simulink model "Pacemaker_images"  (R2022a)
settings: Solver=FixedStepAuto  StartTime=0.0  StopTime=40  FixedStep=1e-3  RelTol=1e-3  EnableMultiTasking=on
undefined symbols (not defined in the file or in its folder): ARP, ATR_Amplitude, ATR_CMP_DETECT, ATR_Pulse_Width, ATR_Sensitivity, D10, D11, D12, D13, D2, D3, D4, D5, D6, D7, D8, D9, Flag, Hecate_delayEnd, Hecate_delayOff, Hecate_delayOn, LRL, Mode, PTA0, PTA1, PTA2, PTB23, PTB9, PTC2, PTC3, PTC4, PTD0, PTD1, PTD2, PTD3, VENT_Amplitude, VENT_CMP_DETECT, VENT_PACE_CTRL, VENT_Pulse_Width, VENT_Sensitivity, VRP
libraries: frdmk64flib x15
settings Model: ExtModeTrigDuration=5  Creator=akshayjacob  LastModifiedBy=fedformi_new
settings DataIOCC: SaveFormat=Array  ReturnWorkspaceOutputs=off
settings OptimizationCC: DefaultParameterBehavior=Inlined  EnhancedBackFolding=on  PassReuseOutputArgsAs=Individual arguments  ZeroExternalMemoryAtStartup=off  ZeroInternalMemoryAtStartup=off  MaxStackSize=64  OptimizeBlockOrder=speed  DifferentSizesBufferReuse=on  OptimizationCustomize=off  EfficientTunableParamExpr=on
settings DebuggingCC: ParameterTunabilityLossMsg=error  UnconnectedInputMsg=warning  UnconnectedOutputMsg=warning  UnconnectedLineMsg=warning
settings HardwareCC: ProdBitPerPointer=32  ProdBitPerSizeT=32  ProdBitPerPtrDiffT=32  ProdLargestAtomicInteger=Long  ProdLargestAtomicFloat=Double  ProdWordSize=32  ProdHWDeviceType=ARM Compatible->ARM Cortex
settings SFSimCC: MATLABDynamicMemAlloc=off
settings RTWCC: SystemTargetFile=ert.tlc  TemplateMakefile=ert_default_tmf  Toolchain=GNU Tools for ARM Embedded Processors  DLArmComputeVersion=19.05
settings CodeAppCC: ForceParamTrailComments=on  IgnoreCustomStorageClasses=off  OperatorAnnotations=on  SimulinkDataObjDesc=on  SFDataObjDesc=on  InsertBlockDesc=on
settings ERTTargetCC: ERTCustomFileTemplate=example_file_process.tlc

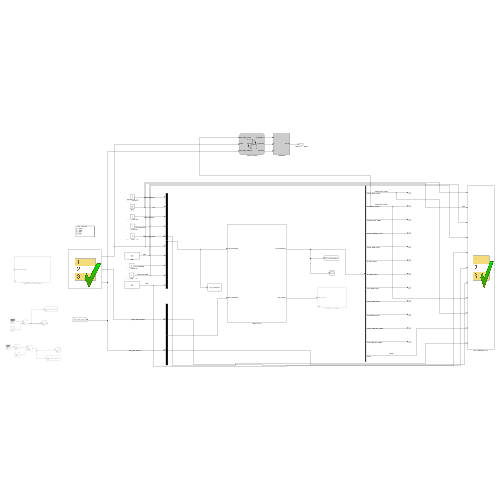
[thumbnail: Simulink's stored preview of the top-level diagram]
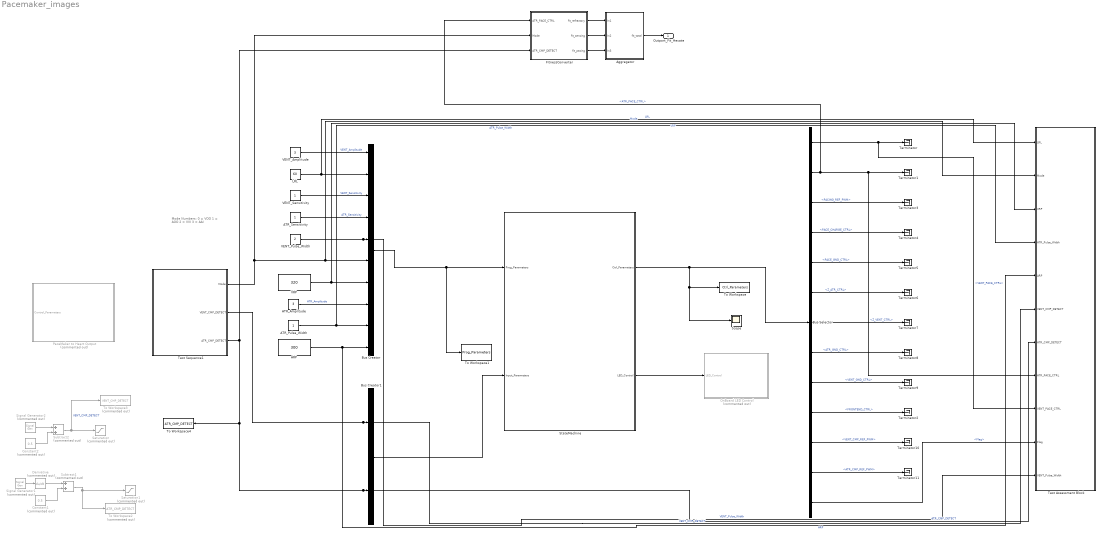
== system Pacemaker_images ==
  note: Mode Numbers:
      |
      | 0 = VOO
      | 1 = AOO
      | 2 = VVI
      | 3 = AAI
  ARP : Constant  Value=300
  ATR_Amplitude : Constant  Value=3
  ATR_Pulse_Width : Constant
  ATR_Sensitivity : Constant
  Aggregator : Subsystem
  Bus Creator : BusCreator  Inputs=VENT_Amplitude,LRL,VENT_Sensitivity,ATR_Sensitivity,VENT_Pulse_Width,Mode,VRP,ATR_Amplitude,ATR_Pulse_Width,ARP
  Bus Creator1 : BusCreator  Inputs=VENT_CMP_DETECT,ATR_CMP_DETECT
  Bus Selector : BusSelector  OutputSignals=VENT_PACE_CTRL,ATR_PACE_CTRL,PACING_REF_PWM,PACE_CHARGE_CTRL,PACE_GND_CTRL,Z_ATR_CTRL,Z_VENT_CTRL,ATR_GND_CTRL,VENT_GND_CTRL,FRONTEND_CTRL,VENT_CMP_REF_PWM,ATR_CMP_REF_PWM,Flag
  Constant1 : Constant  Commented=on  Value=0.5
  Constant2 : Constant  Commented=on  Value=0.5
  Derivative : Derivative  Commented=on
  FitnessConverter : Stateflow chart  TreatAsAtomicUnit=on
  LRL : Constant  Value=60
  OnBoard LED Control : Subsystem  Commented=on
  PaceMaker to Heart Output : Subsystem  Commented=on
  Saturation : Saturate  Commented=on  UpperLimit=1  LowerLimit=0
  Saturation1 : Saturate  Commented=on  UpperLimit=1  LowerLimit=0
  Scope : Scope
  Signal Generator1 : SignalGenerator  Commented=on  Amplitude=1.5  Frequency=1/5
  Signal Generator2 : SignalGenerator  Commented=on  Amplitude=1.5  Frequency=1/5
  StateMachine : Subsystem
  Subtract1 : Sum  Commented=on
  Subtract2 : Sum  Commented=on
  Terminator{,1..11} (12 alike) : Terminator
  Test Assessment Block : Test Sequence  Tag=__SLT_ASMT__  TreatAsAtomicUnit=on
  Test Sequence1 : Test Sequence  TreatAsAtomicUnit=on
  To Workspace : ToWorkspace  VariableName=Ctrl_Parameters  SaveFormat=Timeseries  SampleTime=-1
  To Workspace1 : ToWorkspace  VariableName=Prog_Parameters  SaveFormat=Timeseries  SampleTime=-1
  To Workspace2 : ToWorkspace  Commented=on  VariableName=ATR_CMP_DETECT  SaveFormat=Timeseries  SampleTime=-1
  To Workspace3 : ToWorkspace  Commented=on  VariableName=VENT_CMP_DETECT  SaveFormat=Timeseries  SampleTime=-1
  To Workspace4 : ToWorkspace  VariableName=ATR_CMP_DETECT  SaveFormat=Timeseries  SampleTime=-1
  VENT_Amplitude : Constant  Value=3
  VENT_Pulse_Width : Constant  Value=2
  VENT_Sensitivity : Constant
  VRP : Constant  Value=320
  Outport_Fit_Hecate : Outport
  wires:
  Bus Creator/1 -> To Workspace1/1, StateMachine/1(Prog_Parameters)
  StateMachine/2(LED_Control) -> OnBoard LED Control/1(LED_Control)
  Bus Creator1/1 -> StateMachine/2(Input_Parameters)
  VRP/1 -> Bus Creator/7, Test Assessment Block/3(VRP)  "VRP"
  ATR_Sensitivity/1 -> Bus Creator/4  "ATR_Sensitivity"
  ATR_Pulse_Width/1 -> Bus Creator/9, Test Assessment Block/4(ATR_Pulse_Width)  "ATR_Pulse_Width"
  LRL/1 -> Bus Creator/2, Test Assessment Block/1(LRL)  "LRL"
  ATR_Amplitude/1 -> Bus Creator/8  "ATR_Amplitude"
  ARP/1 -> Bus Creator/10, Test Assessment Block/5(ARP)  "ARP"
  VENT_Sensitivity/1 -> Bus Creator/3  "VENT_Sensitivity"
  VENT_Amplitude/1 -> Bus Creator/1  "VENT_Amplitude"
  VENT_Pulse_Width/1 -> Test Assessment Block/11(VENT_Pulse_Width), Bus Creator/5  "VENT_Pulse_Width"
  Test Sequence1/1(Mode) -> Test Assessment Block/2(Mode), Bus Creator/6, FitnessConverter/2(Mode)  "Mode"
  Subtract1/1 -> Saturation1/1, To Workspace2/1
  Signal Generator2/1 -> Subtract2/1
  Test Sequence1/2(VENT_CMP_DETECT) -> Test Assessment Block/6(VENT_CMP_DETECT), Bus Creator1/1  "VENT_CMP_DETECT"
  Constant1/1 -> Subtract1/2
  Constant2/1 -> Subtract2/2
  Test Sequence1/3(ATR_CMP_DETECT) -> FitnessConverter/3(ATR_CMP_DETECT), To Workspace4/1, Test Assessment Block/7(ATR_CMP_DETECT), Bus Creator1/2  "ATR_CMP_DETECT"
  Subtract2/1 -> Saturation/1, To Workspace3/1  "VENT_CMP_DETECT"
  Derivative/1 -> Subtract1/1
  Signal Generator1/1 -> Derivative/1
  Bus Selector/12 -> Terminator11/1  "<ATR_CMP_REF_PWM>"
  Bus Selector/3 -> Terminator3/1  "<PACING_REF_PWM>"
  Bus Selector/7 -> Terminator7/1  "<Z_VENT_CTRL>"
  Bus Selector/10 -> Terminator2/1  "<FRONTEND_CTRL>"
  Bus Selector/8 -> Terminator8/1  "<ATR_GND_CTRL>"
  StateMachine/1(Ctrl_Parameters) -> Bus Selector/1, Scope/1, To Workspace/1
  Bus Selector/1 -> Test Assessment Block/9(VENT_PACE_CTRL), Terminator/1  "<VENT_PACE_CTRL>"
  Bus Selector/5 -> Terminator5/1  "<PACE_GND_CTRL>"
  Bus Selector/9 -> Terminator9/1  "<VENT_GND_CTRL>"
  Bus Selector/2 -> Test Assessment Block/8(ATR_PACE_CTRL), Terminator1/1, FitnessConverter/1(ATR_PACE_CTRL)  "<ATR_PACE_CTRL>"
  Bus Selector/11 -> Terminator10/1  "<VENT_CMP_REF_PWM>"
  Bus Selector/6 -> Terminator6/1  "<Z_ATR_CTRL>"
  Bus Selector/4 -> Terminator4/1  "<PACE_CHARGE_CTRL>"
  Bus Selector/13 -> Test Assessment Block/10(Flag)  "<Flag>"
  FitnessConverter/1(fit_refractory) -> Aggregator/1(In1)
  FitnessConverter/2(fit_sensing) -> Aggregator/2(In2)
  FitnessConverter/3(fit_pacing) -> Aggregator/3(In3)
  Aggregator/1(fit_total) -> Outport_Fit_Hecate/1

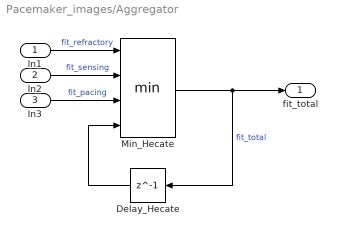
== system Pacemaker_images/Aggregator ==
  In1 : Inport
  In2 : Inport  Port=2
  In3 : Inport  Port=3
  Delay_Hecate : Delay  DelayLength=1  InitialCondition=Inf
  Min_Hecate : MinMax  Inputs=4
  fit_total : Outport
  wires:
  In2/1 -> Min_Hecate/2  "fit_sensing"
  In3/1 -> Min_Hecate/3  "fit_pacing"
  Delay_Hecate/1 -> Min_Hecate/4
  In1/1 -> Min_Hecate/1  "fit_refractory"
  Min_Hecate/1 -> fit_total/1, Delay_Hecate/1  "fit_total"

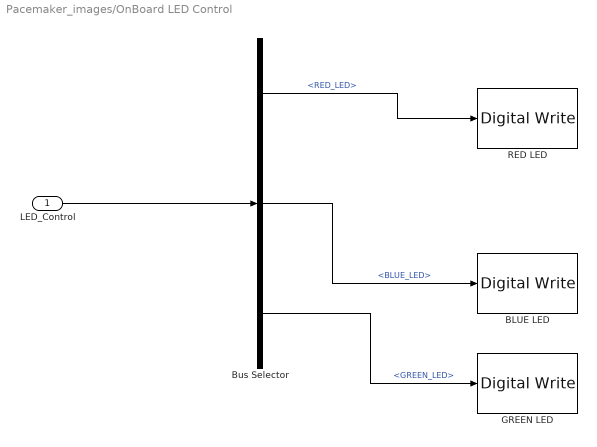
== system Pacemaker_images/OnBoard LED Control ==
  LED_Control : Inport
  BLUE LED : frdmk64flib/Digital Write  Whichpin=BLUE_LED
  Bus Selector : BusSelector  OutputSignals=RED_LED,BLUE_LED,GREEN_LED
  GREEN LED : frdmk64flib/Digital Write  Whichpin=GREEN_LED
  RED LED : frdmk64flib/Digital Write  Whichpin=RED_LED
  wires:
  LED_Control/1 -> Bus Selector/1
  Bus Selector/1 -> RED LED/1  "<RED_LED>"
  Bus Selector/2 -> BLUE LED/1  "<BLUE_LED>"
  Bus Selector/3 -> GREEN LED/1  "<GREEN_LED>"

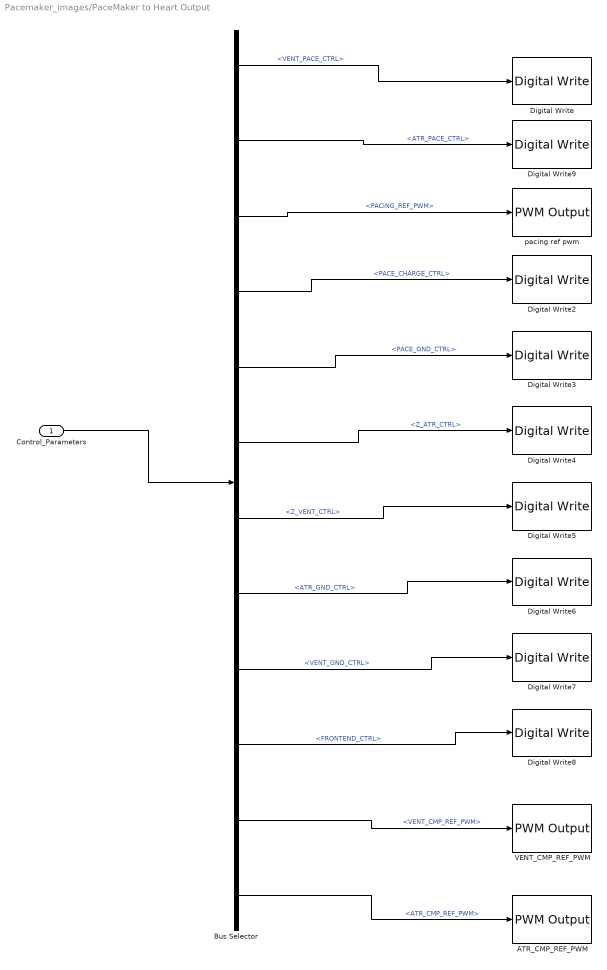
== system Pacemaker_images/PaceMaker to Heart Output ==
  Control_Parameters : Inport
  ATR_CMP_REF_PWM : frdmk64flib/PWM Output  Whichpin=PTC2 (D6)  InitialFrequency=2000  InitialDutyCycle=0
  Bus Selector : BusSelector  OutputSignals=VENT_PACE_CTRL,ATR_PACE_CTRL,PACING_REF_PWM,PACE_CHARGE_CTRL,PACE_GND_CTRL,Z_ATR_CTRL,Z_VENT_CTRL,ATR_GND_CTRL,VENT_GND_CTRL,FRONTEND_CTRL,VENT_CMP_REF_PWM,ATR_CMP_REF_PWM
  Digital Write : frdmk64flib/Digital Write  Whichpin=PTC4 (D9)
  Digital Write2 : frdmk64flib/Digital Write  Whichpin=PTB9 (D2)
  Digital Write3 : frdmk64flib/Digital Write  Whichpin=PTD0 (D10)
  Digital Write4 : frdmk64flib/Digital Write  Whichpin=PTB23 (D4)
  Digital Write5 : frdmk64flib/Digital Write  Whichpin=PTC3 (D7)
  Digital Write6 : frdmk64flib/Digital Write  Whichpin=PTD2 (D11)
  Digital Write7 : frdmk64flib/Digital Write  Whichpin=PTD3 (D12)
  Digital Write8 : frdmk64flib/Digital Write  Whichpin=PTD1 (D13)
  Digital Write9 : frdmk64flib/Digital Write  Whichpin=PTA0 (D8)
  VENT_CMP_REF_PWM : frdmk64flib/PWM Output  Whichpin=PTA1 (D3)  InitialFrequency=2000  InitialDutyCycle=0
  pacing ref pwm : frdmk64flib/PWM Output  Whichpin=PTA2 (D5)  InitialFrequency=2000  InitialDutyCycle=0
  wires:
  Control_Parameters/1 -> Bus Selector/1
  Bus Selector/1 -> Digital Write/1  "<VENT_PACE_CTRL>"
  Bus Selector/3 -> pacing ref pwm/1  "<PACING_REF_PWM>"
  Bus Selector/4 -> Digital Write2/1  "<PACE_CHARGE_CTRL>"
  Bus Selector/5 -> Digital Write3/1  "<PACE_GND_CTRL>"
  Bus Selector/6 -> Digital Write4/1  "<Z_ATR_CTRL>"
  Bus Selector/7 -> Digital Write5/1  "<Z_VENT_CTRL>"
  Bus Selector/8 -> Digital Write6/1  "<ATR_GND_CTRL>"
  Bus Selector/9 -> Digital Write7/1  "<VENT_GND_CTRL>"
  Bus Selector/10 -> Digital Write8/1  "<FRONTEND_CTRL>"
  Bus Selector/2 -> Digital Write9/1  "<ATR_PACE_CTRL>"
  Bus Selector/11 -> VENT_CMP_REF_PWM/1  "<VENT_CMP_REF_PWM>"
  Bus Selector/12 -> ATR_CMP_REF_PWM/1  "<ATR_CMP_REF_PWM>"

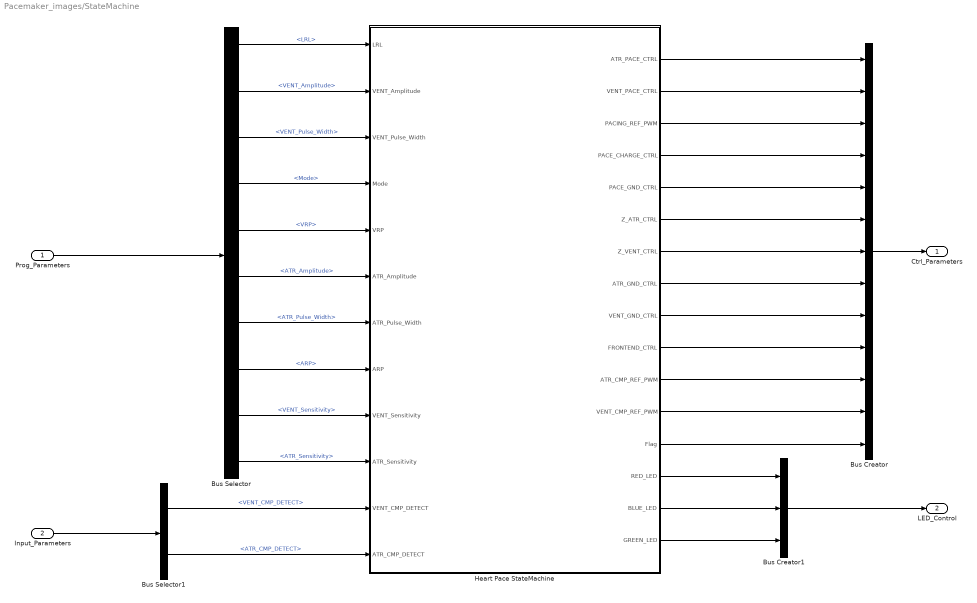
== system Pacemaker_images/StateMachine ==
  Prog_Parameters : Inport
  Input_Parameters : Inport  Port=2
  Bus Creator : BusCreator  Inputs=13
  Bus Creator1 : BusCreator  Inputs=3
  Bus Selector : BusSelector  OutputSignals=LRL,VENT_Amplitude,VENT_Pulse_Width,Mode,VRP,ATR_Amplitude,ATR_Pulse_Width,ARP,VENT_Sensitivity,ATR_Sensitivity
  Bus Selector1 : BusSelector  OutputSignals=VENT_CMP_DETECT,ATR_CMP_DETECT
  Heart Pace StateMachine : Stateflow chart  TreatAsAtomicUnit=on
      settings: PortSchema="{\"entries\":[{\"content\":{\"sides\":[{\"content\":{\"connectorIds\":[\"In1\",\"In2\",\"In3\",\"In4\",\"In5\",\"In6\",\"In7\",\"In8\",\"In9\",\"In10\",\"In11\",\"In12\"]},\"type\":\"ConnectorPlacement.EquallySpacedRectSide\",\"uuid\":\"078f44e2-9792-46c6-9fab-c05fe0916fc5\"},{\"content\":{\"connectorIds\":[\"Out1\",\"Out2\",\"Out3\",\"Out4\",\"Out5\",\"Out6\",\"Out7\",\"Out8\",\"Out9\",\"Out10\",\"Out14\",\"Out15\",\"Out16\",\"Out11\",\"Out12\",\"Out13\"],\"side\":\"RIGHT\"},\"type\":\"ConnectorPlacement.EquallySpacedRectSide\",\"uuid\":\"2df68980-2ea6-42d1-b726-b24978220bfa\"},{\"content\":{\"connectorIds\":[],\"side\":\"TOP\"},\"type\":\"ConnectorPlacement.EquallySpacedRectSide\",\"uuid\":\"4f99418a-e276-4e4c-8fb0-96ffb017fecf\"}]},\"type\":\"ConnectorPlacement.EquallySpacedConnector\",\"uuid\":\"ac4267e7-732c-486f-b9a5-28cca0f40ec4\"}],\"packageUris\":[\"http://schema.mathworks.com/mf0/Connector/R2020b\"],\"version\":\"1.0\"}"
  Ctrl_Parameters : Outport
  LED_Control : Outport  Port=2
  wires:
  Prog_Parameters/1 -> Bus Selector/1
  Bus Selector/1 -> Heart Pace StateMachine/1(LRL)  "<LRL>"
  Bus Selector/2 -> Heart Pace StateMachine/2(VENT_Amplitude)  "<VENT_Amplitude>"
  Bus Selector/3 -> Heart Pace StateMachine/3(VENT_Pulse_Width)  "<VENT_Pulse_Width>"
  Bus Selector/4 -> Heart Pace StateMachine/4(Mode)  "<Mode>"
  Heart Pace StateMachine/1(ATR_PACE_CTRL) -> Bus Creator/1
  Heart Pace StateMachine/2(VENT_PACE_CTRL) -> Bus Creator/2
  Bus Creator/1 -> Ctrl_Parameters/1
  Heart Pace StateMachine/3(PACING_REF_PWM) -> Bus Creator/3
  Heart Pace StateMachine/4(PACE_CHARGE_CTRL) -> Bus Creator/4
  Heart Pace StateMachine/5(PACE_GND_CTRL) -> Bus Creator/5
  Heart Pace StateMachine/6(Z_ATR_CTRL) -> Bus Creator/6
  Heart Pace StateMachine/7(Z_VENT_CTRL) -> Bus Creator/7
  Heart Pace StateMachine/8(ATR_GND_CTRL) -> Bus Creator/8
  Heart Pace StateMachine/9(VENT_GND_CTRL) -> Bus Creator/9
  Heart Pace StateMachine/10(FRONTEND_CTRL) -> Bus Creator/10
  Heart Pace StateMachine/11(RED_LED) -> Bus Creator1/1
  Heart Pace StateMachine/12(BLUE_LED) -> Bus Creator1/2
  Bus Creator1/1 -> LED_Control/1
  Heart Pace StateMachine/13(GREEN_LED) -> Bus Creator1/3
  Input_Parameters/1 -> Bus Selector1/1
  Bus Selector1/1 -> Heart Pace StateMachine/11(VENT_CMP_DETECT)  "<VENT_CMP_DETECT>"
  Bus Selector1/2 -> Heart Pace StateMachine/12(ATR_CMP_DETECT)  "<ATR_CMP_DETECT>"
  Bus Selector/6 -> Heart Pace StateMachine/6(ATR_Amplitude)  "<ATR_Amplitude>"
  Bus Selector/7 -> Heart Pace StateMachine/7(ATR_Pulse_Width)  "<ATR_Pulse_Width>"
  Bus Selector/8 -> Heart Pace StateMachine/8(ARP)  "<ARP>"
  Bus Selector/9 -> Heart Pace StateMachine/9(VENT_Sensitivity)  "<VENT_Sensitivity>"
  Bus Selector/10 -> Heart Pace StateMachine/10(ATR_Sensitivity)  "<ATR_Sensitivity>"
  Heart Pace StateMachine/14(ATR_CMP_REF_PWM) -> Bus Creator/11
  Heart Pace StateMachine/15(VENT_CMP_REF_PWM) -> Bus Creator/12
  Bus Selector/5 -> Heart Pace StateMachine/5(VRP)  "<VRP>"
  Heart Pace StateMachine/16(Flag) -> Bus Creator/13

== stateflow chart Pacemaker_images/Test Assessment Block ==
  state Run
    state AAI
      state AAI_Refractory
        verify(ATR_PACE_CTRL==0)
      state AAI_Sensing
        verify(ATR_PACE_CTRL==0)
      state AAI_Pacing
        verify(ATR_PACE_CTRL==1);
      (default) -> AAI_Refractory
      (junction 475) -> AAI_Refractory
      (junction 494) -> (junction 475)
      AAI_Refractory -> AAI_Sensing : [
          | after(ARP-(ATR_Pulse_Width ...
          | *Flag),msec)
          | ]
      AAI_Sensing -> AAI_Refractory [order 1] : [
          | [(ATR_CMP_DETECT == 1)]
          | ]
      AAI_Sensing -> AAI_Pacing [order 2] : [
          | after(60000/LRL-ARP, msec)
          | ]
      AAI_Pacing -> (junction 494) : [
          | after(ATR_Pulse_Width,msec)
          | ]
    state VVI
      state VVI_REFRACTORY
        verify(VENT_PACE_CTRL==0);
      state VVI_SENSE
        verify(VENT_PACE_CTRL==0);
      state VVI_PACING
        verify(VENT_PACE_CTRL==1);
      (junction 541) -> (junction 535)
      (default) -> VVI_REFRACTORY
      (junction 535) -> VVI_REFRACTORY
      VVI_REFRACTORY -> VVI_SENSE : [
          | after(VRP - (VENT_Pulse_Width * Flag-1),msec)
          | ]
      VVI_SENSE -> VVI_REFRACTORY [order 2] : [
          | VENT_CMP_DETECT == 1
          | ]
      VVI_SENSE -> VVI_PACING [order 1] : [
          | after(60000/LRL - VRP, msec)
          | ]
      VVI_PACING -> (junction 541) : [
          | after(VENT_Pulse_Width,msec)
          | ]
    state default
    (junction 517) -> (junction 520) [order 2]
    (junction 407) -> (junction 516) [order 2]
    Run -> (junction 407)
    (junction 407) -> (junction 390) [order 1] : [Mode == 3
        | ]
    (junction 516) -> (junction 418) [order 2]
    (junction 390) -> AAI [order 1] : [~in(Run.AAI)]
    (junction 390) -> (junction 393) [order 2]
    (default) -> (junction 407)
    (junction 516) -> (junction 517) [order 1] : [Mode ==2
        | ]
    (junction 517) -> VVI [order 1] : [~in(Run.VVI)]
    (junction 418) -> (junction 419)
    (junction 419) -> default [order 1] : [~in(Run.default)]
    (junction 419) -> (junction 422) [order 2]
  (default) -> Run
  data: LRL input double size=[1]; Mode input double size=[1]; VRP input size=[1]; ATR_Pulse_Width input double size=[1]; ARP input size=[1]; VENT_CMP_DETECT input size=[1, 1]; ATR_CMP_DETECT input size=[1, 1]; ATR_PACE_CTRL input double size=[1]; VENT_PACE_CTRL input double size=[1]; Flag input; VENT_Pulse_Width input

== stateflow chart Pacemaker_images/Test Sequence1 ==
  settings: updateMethod=DISCRETE  sampleTime=0.001
  state Initialize
    %. . .
    ATR_CMP_DETECT=false;
  state AAI_Mode_3
    Mode=3;
    state AAI_Mode_3_OFF
      ATR_CMP_DETECT=false;
    state AAI_Mode_3_ON
      ATR_CMP_DETECT=true;
    (default) -> AAI_Mode_3_OFF
    AAI_Mode_3_OFF -> AAI_Mode_3_ON : [
        | after(3+...
        | Hecate_delayOn,sec)
        | ]
    AAI_Mode_3_ON -> AAI_Mode_3_OFF : [
        | after(1+...
        | Hecate_delayOff,sec)
        | ]
  state END
    ATR_CMP_DETECT=false;
  (default) -> Initialize
  Initialize -> AAI_Mode_3 : [
      | true
      | ]
  AAI_Mode_3 -> END : [
      | after(20+...
      | Hecate_delayEnd,sec)
      | ]
  data: Mode output double size=[1]; VENT_CMP_DETECT output boolean size=[1, 1]; ATR_CMP_DETECT output boolean size=[1, 1]; Hecate_delayEnd parameter; Hecate_delayOn parameter; Hecate_delayOff parameter

== stateflow chart Pacemaker_images/FitnessConverter ==
  state Run
    fit_refractory = Inf;
    fit_sensing = Inf;
    fit_pacing = Inf;
    state default
      fit_refractory = Inf;
      fit_sensing = Inf;
      fit_pacing = Inf;
    state AAI
      fit_refractory = Inf;
      fit_sensing = Inf;
      fit_pacing = Inf;
      state AAI_Refractory
        fit_refractory = ...
        abs(ATR_PACE_CTRL-(0));
        fit_sensing = Inf;
        fit_pacing = Inf;
      state AAI_Sensing
        fit_refractory = Inf;
        fit_sensing = ...
        abs(ATR_PACE_CTRL-(0));
        fit_pacing = Inf;
      state AAI_Pacing
        fit_refractory = Inf;
        fit_sensing = Inf;
        fit_pacing = ...
        abs(ATR_PACE_CTRL-(1));
      AAI_Sensing -> AAI_Refractory [order 1] : [[(ATR_CMP_DETECT == 1)]]
      (default) -> AAI_Refractory
      AAI_Refractory -> AAI_Sensing : [after(ARP-(ATR_Pulse_Width ...
          | *Flag),msec)]
      AAI_Sensing -> AAI_Pacing [order 2] : [after(60000/LRL-ARP, msec)]
      AAI_Pacing -> AAI_Refractory : [after(ATR_Pulse_Width,msec)]
    state VVI
      fit_refractory = Inf;
      fit_sensing = Inf;
      fit_pacing = Inf;
      state VVI_REFRACTORY
        fit_refractory = Inf;
        fit_sensing = Inf;
        fit_pacing = Inf;
      state VVI_SENSE
        fit_refractory = Inf;
        fit_sensing = Inf;
        fit_pacing = Inf;
      state VVI_PACING
        fit_refractory = Inf;
        fit_sensing = Inf;
        fit_pacing = Inf;
      (default) -> VVI_REFRACTORY
      VVI_SENSE -> VVI_REFRACTORY [order 2] : [VENT_CMP_DETECT == 1]
      VVI_PACING -> VVI_REFRACTORY : [after(VENT_Pulse_Width,msec)]
      VVI_SENSE -> VVI_PACING [order 1] : [after(60000/LRL - VRP, msec)]
      VVI_REFRACTORY -> VVI_SENSE : [after(VRP - (VENT_Pulse_Width * Flag-1),msec)]
    default -> (junction 48) : [(Mode==2)|(Mode==3)]
    (default) -> (junction 48)
    (junction 48) -> default [order 3]
    AAI -> (junction 48) : [~(Mode==2)]
    (junction 48) -> VVI [order 2] : [Mode==3]
    VVI -> (junction 48) : [(Mode==2)|~(Mode==3)]
    (junction 48) -> AAI [order 1] : [Mode==2]
  (default) -> Run
  data: fit_refractory output; ATR_PACE_CTRL input; Mode input; LRL parameter; VRP parameter; ATR_Pulse_Width parameter; ARP parameter; VENT_CMP_DETECT parameter; VENT_PACE_CTRL parameter; Flag parameter; VENT_Pulse_Width parameter; fit_sensing output; fit_pacing output; ATR_CMP_DETECT input

== stateflow chart Pacemaker_images/StateMachine/Heart Pace StateMachine ==
  state VOO_ChargingState
    entry:
    ATR_PACE_CTRL = 0;
    VENT_PACE_CTRL = 0;
    PACING_REF_PWM = VENT_Amplitude/5*100
    PACE_CHARGE_CTRL = 1;
    PACE_GND_CTRL = 1;
    Z_ATR_CTRL = 0;
    Z_VENT_CTRL = 0;
    ATR_GND_CTRL = 0;
    VENT_GND_CTRL = 1;
    BLUE_LED = 0;
    RED_LED = 1;
  state VOO_Pacing
    entry:
    PACE_CHARGE_CTRL = 0;
    PACE_GND_CTRL = 1;
    ATR_GND_CTRL = 0;
    ATR_PACE_CTRL = 0;
    Z_ATR_CTRL = 0;
    Z_VENT_CTRL =0;
    VENT_PACE_CTRL = 1;
    VENT_GND_CTRL = 0;
    PACING_REF_PWM = VENT_Amplitude/5*100;
    BLUE_LED=1;
    RED_LED=0;
  state AOO_ChargingState
    entry:
    ATR_PACE_CTRL = 0;
    VENT_PACE_CTRL = 0;
    PACING_REF_PWM = ATR_Amplitude/5*100
    PACE_CHARGE_CTRL = 1;
    PACE_GND_CTRL = 1;
    Z_ATR_CTRL = 0;
    Z_VENT_CTRL = 0;
    ATR_GND_CTRL = 1;
    VENT_GND_CTRL = 0;
    BLUE_LED = 0;
    RED_LED = 1;
  state AOO_Pacing
    entry:
    PACE_CHARGE_CTRL = 0;
    PACE_GND_CTRL = 1;
    ATR_GND_CTRL = 0;
    ATR_PACE_CTRL = 1;
    Z_ATR_CTRL = 0;
    Z_VENT_CTRL =0;
    VENT_PACE_CTRL = 0;
    VENT_GND_CTRL = 0;
    PACING_REF_PWM = ATR_Amplitude/5*100;
    BLUE_LED=1;
    RED_LED=0;
  state MAIN
    entry:
    PACE_CHARGE_CTRL = 0;
    VENT_PACE_CTRL = 0;
    ATR_PACE_CTRL = 0;
    PACE_GND_CTRL = 0;
    ATR_GND_CTRL = 0;
    VENT_GND_CTRL = 0;
    Z_ATR_CTRL = 0;
    Z_VENT_CTRL = 0;
    FRONTEND_CTRL = 0;
    RED_LED = 0;
    BLUE_LED=0;
    Flag = 0;
  state VVI_Sensing
    entry:
    BLUE_LED = 0;
    RED_LED = 0;
    GREEN_LED = 1;
    FRONTEND_CTRL = 1;
    Flag = 0;
  state VVI_Refactory
    entry:
    ATR_PACE_CTRL = 0;
    VENT_PACE_CTRL = 0;
    PACING_REF_PWM = VENT_Amplitude/5*100;
    PACE_CHARGE_CTRL = 1;
    PACE_GND_CTRL = 1;
    Z_ATR_CTRL = 0;
    Z_VENT_CTRL = 0;
    ATR_GND_CTRL = 0;
    VENT_GND_CTRL = 1;
    FRONTEND_CTRL = 1;
    VENT_CMP_REF_PWM = VENT_Sensitivity/5*100;
    BLUE_LED = 0;
    RED_LED = 1;
    GREEN_LED = 0;
  state VVI_Pacing
    entry:
    FRONTEND_CTRL = 0;
    PACE_CHARGE_CTRL = 0;
    PACE_GND_CTRL = 1;
    ATR_GND_CTRL = 0;
    ATR_PACE_CTRL = 0;
    Z_ATR_CTRL = 0;
    Z_VENT_CTRL =0;
    VENT_PACE_CTRL = 1;
    VENT_GND_CTRL = 0;
    PACING_REF_PWM = VENT_Amplitude/5*100;
    BLUE_LED = 1;
    RED_LED = 0;
    GREEN_LED = 0;
    Flag = 1;
  state AAI_Sensing
    entry:
    BLUE_LED = 0;
    RED_LED = 0;
    GREEN_LED = 1;
    Flag = 0;
  note: Subtract PW from this based on previous event
      | -sense heart rate: dont (no pulsewith done by pacemaker)
      | -pulsed rate: subtract PW
      |  vrp-(pulsewith*flag)
  state AAI_Refactory
    entry:
    ATR_PACE_CTRL = 0;
    VENT_PACE_CTRL = 0;
    PACING_REF_PWM = ATR_Amplitude/5*100;
    PACE_CHARGE_CTRL = 1;
    PACE_GND_CTRL = 1;
    Z_ATR_CTRL = 0;
    Z_VENT_CTRL = 0;
    ATR_GND_CTRL = 1;
    VENT_GND_CTRL = 0;
    FRONTEND_CTRL = 1;
    ATR_CMP_REF_PWM= ATR_Sensitivity/5*100;
    BLUE_LED = 0;
    RED_LED = 1;
    GREEN_LED = 1;
  state AAI_Pacing
    entry:
    FRONTEND_CTRL = 0;
    PACE_CHARGE_CTRL = 0;
    PACE_GND_CTRL = 1;
    ATR_GND_CTRL = 0;
    ATR_PACE_CTRL = 1;
    Z_ATR_CTRL = 0;
    Z_VENT_CTRL =0;
    VENT_PACE_CTRL = 0;
    VENT_GND_CTRL = 0;
    PACING_REF_PWM = ATR_Amplitude/5*100;
    BLUE_LED = 1;
    RED_LED = 0;
    GREEN_LED = 0;
    Flag = 1;
  VOO_ChargingState -> VOO_Pacing : after((60000/LRL) - VENT_Pulse_Width,msec)
  MAIN -> VOO_ChargingState [order 1] : [Mode == 0]
  VOO_Pacing -> VOO_ChargingState : after(VENT_Pulse_Width, msec)
  (default) -> MAIN
  AOO_ChargingState -> AOO_Pacing : after((60000/LRL) - ATR_Pulse_Width,msec)
  MAIN -> AOO_ChargingState [order 4] : [Mode == 1]
  AOO_Pacing -> AOO_ChargingState : after(ATR_Pulse_Width, msec)
  MAIN -> VVI_Refactory [order 2] : [Mode == 2]
  MAIN -> AAI_Refactory [order 3] : [Mode==3]
  VVI_Refactory -> VVI_Sensing : after(VRP - (VENT_Pulse_Width * Flag),msec)
  VVI_Sensing -> VVI_Pacing [order 2] : after(60000/LRL - VRP, msec)
  VVI_Sensing -> VVI_Refactory [order 1] : [(VENT_CMP_DETECT == 1)]
  VVI_Pacing -> VVI_Refactory : after(VENT_Pulse_Width,msec)
  AAI_Refactory -> AAI_Sensing : after(ARP  - (ATR_Pulse_Width * Flag),msec)
  AAI_Sensing -> AAI_Pacing [order 2] : after(60000/LRL - ARP, msec)
  AAI_Sensing -> AAI_Refactory [order 1] : [ATR_CMP_DETECT >= 1]
  AAI_Pacing -> AAI_Refactory : after(ATR_Pulse_Width,msec)
  data: LRL input; VENT_Amplitude input; VENT_Pulse_Width input; Mode input; ATR_PACE_CTRL output; VENT_PACE_CTRL output; PACING_REF_PWM output; PACE_CHARGE_CTRL output; PACE_GND_CTRL output; Z_ATR_CTRL output; Z_VENT_CTRL output; ATR_GND_CTRL output; VENT_GND_CTRL output; FRONTEND_CTRL output; RED_LED output =0; BLUE_LED output; VRP input; ATR_Amplitude input; ATR_Pulse_Width input; ARP input; VENT_Sensitivity input; ATR_Sensitivity input; GREEN_LED output; VENT_CMP_DETECT input; ATR_CMP_DETECT input; ATR_CMP_REF_PWM output; VENT_CMP_REF_PWM output; Flag output
